simulink model "Model_14Bus_Microgrid_R2018"  (R2018b)
settings: Solver=ode23tb  StartTime=0.0  StopTime=0.35  MaxStep=1e-2  RelTol=1e-3
InitFcn:
  | Set_parameters_R2018
StopFcn:
  | Save_Data;
  | Graphics;
values from neighbouring files (symbols this model uses):
  Clink = Ceq*2    (= 0.217013888889)    [Set_parameters_R2017b.m]    (also in Set_parameters_R2018.m)
  dis1 = 0.15    [Set_parameters_R2017b.m]    (also in Set_parameters_R2018.m)
  dis10 = 6    [Set_parameters_R2017b.m]    (also in Set_parameters_R2018.m)
  dis11 = 3    [Set_parameters_R2017b.m]    (also in Set_parameters_R2018.m)
  dis12 = 6    [Set_parameters_R2017b.m]    (also in Set_parameters_R2018.m)
  dis13 = 3    [Set_parameters_R2017b.m]    (also in Set_parameters_R2018.m)
  dis14 = 2    [Set_parameters_R2017b.m]    (also in Set_parameters_R2018.m)
  dis2 = 0.2    [Set_parameters_R2017b.m]    (also in Set_parameters_R2018.m)
  dis3 = 0.15    [Set_parameters_R2017b.m]    (also in Set_parameters_R2018.m)
  dis4 = 0.4    [Set_parameters_R2017b.m]    (also in Set_parameters_R2018.m)
  dis5 = 0.4    [Set_parameters_R2017b.m]    (also in Set_parameters_R2018.m)
  dis6 = 0.4    [Set_parameters_R2017b.m]    (also in Set_parameters_R2018.m)
  dis7 = 0.1    [Set_parameters_R2017b.m]    (also in Set_parameters_R2018.m)
  dis8 = 2    [Set_parameters_R2017b.m]    (also in Set_parameters_R2018.m)
  dis9 = 6    [Set_parameters_R2017b.m]    (also in Set_parameters_R2018.m)
  Fc = 33 * Fnom    (= 1980)    [Set_parameters_R2017b.m]    (also in Set_parameters_R2018.m)
  Fnom = 60    [Main_DC_MG.m]    (also in Set_parameters_R2017b.m; Set_parameters_R2018.m)
  Increment_MPPT = 0.01    [Set_parameters_R2017b.m]    (also in Set_parameters_R2018.m)
  Ki_Ireg = 20    [Set_parameters_R2017b.m]    (also in Set_parameters_R2018.m)
  Ki_VDCreg = 400    [Set_parameters_R2017b.m]    (also in Set_parameters_R2018.m)
  Kp_Ireg = 0.3    [Set_parameters_R2017b.m]    (also in Set_parameters_R2018.m)
  Kp_VDCreg = 2    [Set_parameters_R2017b.m]    (also in Set_parameters_R2018.m)
  LimitL_Ireg = -1.5    [Set_parameters_R2017b.m]    (also in Set_parameters_R2018.m)
  LimitL_VDCreg = -1.5    [Set_parameters_R2017b.m]    (also in Set_parameters_R2018.m)
  Limits_MPPT = [ 583 357 ]    [Set_parameters_R2017b.m]    (also in Set_parameters_R2018.m)
  LimitU_Ireg = 1.5    [Set_parameters_R2017b.m]    (also in Set_parameters_R2018.m)
  LimitU_VDCreg = 1.5    [Set_parameters_R2017b.m]    (also in Set_parameters_R2018.m)
  P_Load_2 = S_Load_2* PF_Load_2    (= 36000)    [Set_parameters_R2017b.m]    (also in Set_parameters_R2018.m)
  P_Load_3 = S_Load_3* PF_Load_3    (= 25500)    [Set_parameters_R2017b.m]    (also in Set_parameters_R2018.m)
  Pnom = 1e6    (= 1000000)    [Set_parameters_R2017b.m]    (also in Set_parameters_R2018.m)
  Pnom_T1 = 1.5e6    (= 1500000)    [Set_parameters_R2017b.m]    (also in Set_parameters_R2018.m)
  Pnom_T2 = 1.5e6    (= 1500000)    [Set_parameters_R2017b.m]    (also in Set_parameters_R2018.m)
  Pnom_T3 = 4e6    (= 4000000)    [Set_parameters_R2017b.m]    (also in Set_parameters_R2018.m)
  Pnom_xfo = Pnom    (= 1000000)    [Set_parameters_R2017b.m]    (also in Set_parameters_R2018.m)
  Ql_Load_2 = S_Load_2 * sin(acos(PF_Load_2))    [Set_parameters_R2017b.m]    (also in Set_parameters_R2018.m)
  Ql_Load_3 = S_Load_3 * sin(acos(PF_Load_3))    [Set_parameters_R2017b.m]    (also in Set_parameters_R2018.m)
  R_Load_9 = (Vnom_prim * 1.35)^2 / P_Load_9    (= 1084.6153125)    [Set_parameters_R2017b.m]    (also in Set_parameters_R2018.m)
  R_Load_DC = Vnom_DC^2/ P_Load_DC    (= 45)    [Main_DC_MG.m]    (also in Set_parameters_R2017b.m; Set_parameters_R2018.m)
  Rl = 0.394    [Set_parameters_R2017b.m]    (also in Set_parameters_R2018.m)
  Rls = 0.198    [Set_parameters_R2017b.m]    (also in Set_parameters_R2018.m)
  Ts = Ts_Power    (= 5.05050505051e-06)    [Main_DC_MG.m]    (also in Set_parameters_R2017b.m; Set_parameters_R2018.m)
  Ts_Control = 10*Ts_Power    (= 5.05050505051e-05)    [Main_DC_MG.m]    (also in Set_parameters_R2017b.m; Set_parameters_R2018.m)
  Ts_Power = 1/(33*Fnom)/100    (= 5.05050505051e-06)    [Main_DC_MG.m]    (also in Set_parameters_R2017b.m; Set_parameters_R2018.m)
  V1_LL_T3 = 69e3    (= 69000)    [Set_parameters_R2017b.m]    (also in Set_parameters_R2018.m)
  Vf = 0    [Set_parameters_R2017b.m]    (also in Set_parameters_R2018.m)
  Vfd = 0    [Set_parameters_R2017b.m]    (also in Set_parameters_R2018.m)
  Vnom_DC = 300    [Main_DC_MG.m]    (also in Set_parameters_R2017b.m; Set_parameters_R2018.m)
  Vnom_dc = 480    [Set_parameters_R2017b.m]    (also in Set_parameters_R2018.m)
  Vnom_Diesel = 2.4e3    (= 2400)    [Set_parameters_R2017b.m]    (also in Set_parameters_R2018.m)
  Vnom_prim = 13.8e3    (= 13800)    [Set_parameters_R2017b.m]    (also in Set_parameters_R2018.m)
  Vnom_sec = 220    [Set_parameters_R2017b.m]    (also in Set_parameters_R2018.m)
  Vnom_ter_AC_DC = 150    [Set_parameters_R2017b.m]    (also in Set_parameters_R2018.m)
  Xl = 0.1168    [Set_parameters_R2017b.m]    (also in Set_parameters_R2018.m)
  Xls = 0.1089    [Set_parameters_R2017b.m]    (also in Set_parameters_R2018.m)
undefined symbols (not defined in the file or in its folder): D1, Delta, Hydride, Ion, Lithium, max_min, Metal, Nickel, RL, RLff, sigbuilder_block
libraries: powerlib x202, powerlib_meascontrol x152, simulink x14, powerlib_extras x14, electricdrivelib x4, re_lib x2
(part 7 of 10)

== system Model_14Bus_Microgrid_R2018/Load_1/Power Factor Block1 ==
  Vabc : Inport
  Iabc : Inport  Port=2
  Complex to Magnitude-Angle : ComplexToMagnitudeAngle
  Mux : Mux  Inputs=2
  Mux1 : Mux  Inputs=2
  Power : powerlib_meascontrol/Measurements/Power  Freq=Freq  Vinit=Vinit  Iinit=Iinit  Ts=Ts
      settings: SourceProductName=Simscape Electrical
  RMS3 : powerlib_meascontrol/Measurements/RMS  TrueRMS=on  Freq=60  RMSInit=0  Ts=0
      settings: SourceProductName=Simscape Electrical
  RMS4 : powerlib_meascontrol/Measurements/RMS  TrueRMS=on  Freq=60  RMSInit=0  Ts=0
      settings: SourceProductName=Simscape Electrical
  Real-Imag to Complex : RealImagToComplex
  Terminator : Terminator
  compara : Gain  SaturateOnIntegerOverflow=on  OutDataTypeStr=Inherit: Same as input  ParamDataTypeStr=Inherit: Same as input
  cos(theta) : Trigonometry  Operator=cos
  Pabc : Outport
  Qabc : Outport  Port=2
  Vabc y Vabc (rms) : Outport  Port=3
  Iabc y Iabc (rms) : Outport  Port=4
  "PFabc " : Outport  Port=5
  wires:
  Power/1 -> Pabc/1, Real-Imag to Complex/1
  Power/2 -> Qabc/1, Real-Imag to Complex/2
  Complex to Magnitude-Angle/2 -> cos(theta)/1
  Real-Imag to Complex/1 -> Complex to Magnitude-Angle/1
  cos(theta)/1 -> "PFabc "/1
  Complex to Magnitude-Angle/1 -> Terminator/1
  Iabc/1 -> RMS4/1, compara/1, Power/2
  RMS4/1 -> Mux1/2
  Mux1/1 -> Iabc y Iabc (rms)/1
  Mux/1 -> Vabc y Vabc (rms)/1
  Vabc/1 -> Power/1, Mux/2, RMS3/1
  compara/1 -> Mux1/1
  RMS3/1 -> Mux/1

== system Model_14Bus_Microgrid_R2018/Load_2/Power Factor Block1 ==
  Vabc : Inport
  Iabc : Inport  Port=2
  Complex to Magnitude-Angle : ComplexToMagnitudeAngle
  Mux : Mux  Inputs=2
  Mux1 : Mux  Inputs=2
  Power : powerlib_meascontrol/Measurements/Power  Freq=Freq  Vinit=Vinit  Iinit=Iinit  Ts=Ts
      settings: SourceProductName=Simscape Electrical
  RMS3 : powerlib_meascontrol/Measurements/RMS  TrueRMS=on  Freq=60  RMSInit=0  Ts=0
      settings: SourceProductName=Simscape Electrical
  RMS4 : powerlib_meascontrol/Measurements/RMS  TrueRMS=on  Freq=60  RMSInit=0  Ts=0
      settings: SourceProductName=Simscape Electrical
  Real-Imag to Complex : RealImagToComplex
  Terminator : Terminator
  compara : Gain  SaturateOnIntegerOverflow=on  OutDataTypeStr=Inherit: Same as input  ParamDataTypeStr=Inherit: Same as input
  cos(theta) : Trigonometry  Operator=cos
  Pabc : Outport
  Qabc : Outport  Port=2
  Vabc y Vabc (rms) : Outport  Port=3
  Iabc y Iabc (rms) : Outport  Port=4
  "PFabc " : Outport  Port=5
  wires:
  Power/1 -> Pabc/1, Real-Imag to Complex/1
  Power/2 -> Qabc/1, Real-Imag to Complex/2
  Complex to Magnitude-Angle/2 -> cos(theta)/1
  Real-Imag to Complex/1 -> Complex to Magnitude-Angle/1
  cos(theta)/1 -> "PFabc "/1
  Complex to Magnitude-Angle/1 -> Terminator/1
  Iabc/1 -> RMS4/1, compara/1, Power/2
  RMS4/1 -> Mux1/2
  Mux1/1 -> Iabc y Iabc (rms)/1
  Mux/1 -> Vabc y Vabc (rms)/1
  Vabc/1 -> Power/1, Mux/2, RMS3/1
  compara/1 -> Mux1/1
  RMS3/1 -> Mux/1

== system Model_14Bus_Microgrid_R2018/Load_3/Power Factor Block1 ==
  Vabc : Inport
  Iabc : Inport  Port=2
  Complex to Magnitude-Angle : ComplexToMagnitudeAngle
  Mux : Mux  Inputs=2
  Mux1 : Mux  Inputs=2
  Power : powerlib_meascontrol/Measurements/Power  Freq=Freq  Vinit=Vinit  Iinit=Iinit  Ts=Ts
      settings: SourceProductName=Simscape Electrical
  RMS3 : powerlib_meascontrol/Measurements/RMS  TrueRMS=on  Freq=60  RMSInit=0  Ts=0
      settings: SourceProductName=Simscape Electrical
  RMS4 : powerlib_meascontrol/Measurements/RMS  TrueRMS=on  Freq=60  RMSInit=0  Ts=0
      settings: SourceProductName=Simscape Electrical
  Real-Imag to Complex : RealImagToComplex
  Terminator : Terminator
  compara : Gain  SaturateOnIntegerOverflow=on  OutDataTypeStr=Inherit: Same as input  ParamDataTypeStr=Inherit: Same as input
  cos(theta) : Trigonometry  Operator=cos
  Pabc : Outport
  Qabc : Outport  Port=2
  Vabc y Vabc (rms) : Outport  Port=3
  Iabc y Iabc (rms) : Outport  Port=4
  "PFabc " : Outport  Port=5
  wires:
  Power/1 -> Pabc/1, Real-Imag to Complex/1
  Power/2 -> Qabc/1, Real-Imag to Complex/2
  Complex to Magnitude-Angle/2 -> cos(theta)/1
  Real-Imag to Complex/1 -> Complex to Magnitude-Angle/1
  cos(theta)/1 -> "PFabc "/1
  Complex to Magnitude-Angle/1 -> Terminator/1
  Iabc/1 -> RMS4/1, compara/1, Power/2
  RMS4/1 -> Mux1/2
  Mux1/1 -> Iabc y Iabc (rms)/1
  Mux/1 -> Vabc y Vabc (rms)/1
  Vabc/1 -> Power/1, Mux/2, RMS3/1
  compara/1 -> Mux1/1
  RMS3/1 -> Mux/1

== system Model_14Bus_Microgrid_R2018/Load_4/Power Factor Block1 ==
  Vabc : Inport
  Iabc : Inport  Port=2
  Complex to Magnitude-Angle : ComplexToMagnitudeAngle
  Mux : Mux  Inputs=2
  Mux1 : Mux  Inputs=2
  Power : powerlib_meascontrol/Measurements/Power  Freq=Freq  Vinit=Vinit  Iinit=Iinit  Ts=Ts
      settings: SourceProductName=Simscape Electrical
  RMS3 : powerlib_meascontrol/Measurements/RMS  TrueRMS=on  Freq=60  RMSInit=0  Ts=0
      settings: SourceProductName=Simscape Electrical
  RMS4 : powerlib_meascontrol/Measurements/RMS  TrueRMS=on  Freq=60  RMSInit=0  Ts=0
      settings: SourceProductName=Simscape Electrical
  Real-Imag to Complex : RealImagToComplex
  Terminator : Terminator
  compara : Gain  SaturateOnIntegerOverflow=on  OutDataTypeStr=Inherit: Same as input  ParamDataTypeStr=Inherit: Same as input
  cos(theta) : Trigonometry  Operator=cos
  Pabc : Outport
  Qabc : Outport  Port=2
  Vabc y Vabc (rms) : Outport  Port=3
  Iabc y Iabc (rms) : Outport  Port=4
  "PFabc " : Outport  Port=5
  wires:
  Power/1 -> Pabc/1, Real-Imag to Complex/1
  Power/2 -> Qabc/1, Real-Imag to Complex/2
  Complex to Magnitude-Angle/2 -> cos(theta)/1
  Real-Imag to Complex/1 -> Complex to Magnitude-Angle/1
  cos(theta)/1 -> "PFabc "/1
  Complex to Magnitude-Angle/1 -> Terminator/1
  Iabc/1 -> RMS4/1, compara/1, Power/2
  RMS4/1 -> Mux1/2
  Mux1/1 -> Iabc y Iabc (rms)/1
  Mux/1 -> Vabc y Vabc (rms)/1
  Vabc/1 -> Power/1, Mux/2, RMS3/1
  compara/1 -> Mux1/1
  RMS3/1 -> Mux/1

== system Model_14Bus_Microgrid_R2018/Resource1/Irradiance Temp Demand Max ==
  Demux : Demux  Tag=STV Demux  Outputs=2
  FromWs : FromWorkspace  Tag=STV FromWs  VariableName=tuvar  SampleTime=0
      SigBuilderData=|
      | common.afterFinalStr = 'Extrapolate'
      | common.sampleTime = '0'
      | dataSet(1).timeRange = [0 2]
      | dataSet(1).name = 'Constant Irradiance'
      | dataSet(2).timeRange = [0 2]
      | dataSet(2).name = 'Step Irradiance'
      | dataSet(3).timeRange = [0 3]
      | dataSet(3).name = 'Ramp-up/down Irradiance'
      | sbobj.Groups(1).Name = 'Constant Irradiance'
      | sbobj.Groups(1).Signals(1).Name = 'Ir'
      | sbobj.Groups(1).Signals(1).XData = [0 2]
      | sbobj.Groups(1).Signals(1).YData = [1000 1000]
      | sbobj.Groups(1).Signals(2).Name = 'Temp'
      | sbobj.Groups(1).Signals(2).XData = [0 1 1 2]
      | sbobj.Groups(1).Signals(2).YData = [0 0 1 1]
      | sbobj.Groups(1).TimeRange = [0 2]
      | sbobj.Groups(2).Name = 'Step Irradiance'
      | sbobj.Groups(2).Signals(1).Name = 'Ir'
      | sbobj.Groups(2).Signals(1).XData = [0 0.252 0.252 2]
      | sbobj.Groups(2).Signals(1).YData = [600 600 1000 1000]
      | sbobj.Groups(2).Signals(2).Name = 'Temp'
      | sbobj.Groups(2).Signals(2).XData = [0 1 1 2]
      | sbobj.Groups(2).Signals(2).YData = [0 0 1 1]
      | sbobj.Groups(2).TimeRange = [0 2]
      | sbobj.Groups(3).Name = 'Ramp-up/down Irradiance'
      | sbobj.Groups(3).Signals(1).Name = 'Ir'
      | sbobj.Groups(3).Signals(1).XData = [0 0.785 1.7 2.28 3]
      | sbobj.Groups(3).Signals(1).YData = [1000 999.538235294 999 999.446153846 1000]
      | sbobj.Groups(3).Signals(2).Name = 'Temp'
      | sbobj.Groups(3).Signals(2).XData = [0 2 2.1 3]
      | sbobj.Groups(3).Signals(2).YData = [25 25 25 25]
      | sbobj.Groups(3).TimeRange = [0 3]
  Ir : Outport  Tag=STV Outport
  Temp : Outport  Tag=STV Outport  Port=2
  wires:
  Demux/1 -> Ir/1
  FromWs/1 -> Demux/1
  Demux/2 -> Temp/1

== system Model_14Bus_Microgrid_R2018/Resources/Irradiance Temp Demand Max ==
  Demux : Demux  Tag=STV Demux  Outputs=2
  FromWs : FromWorkspace  Tag=STV FromWs  VariableName=tuvar  SampleTime=0
      SigBuilderData=|
      | common.afterFinalStr = 'Extrapolate'
      | common.sampleTime = '0'
      | dataSet(1).timeRange = [0 2]
      | dataSet(1).name = 'Constant Irradiance'
      | dataSet(2).timeRange = [0 2]
      | dataSet(2).name = 'Step Irradiance'
      | dataSet(3).timeRange = [0 3]
      | dataSet(3).name = 'Ramp-up/down Irradiance'
      | sbobj.Groups(1).Name = 'Constant Irradiance'
      | sbobj.Groups(1).Signals(1).Name = 'Ir'
      | sbobj.Groups(1).Signals(1).XData = [0 2]
      | sbobj.Groups(1).Signals(1).YData = [1000 1000]
      | sbobj.Groups(1).Signals(2).Name = 'Temp'
      | sbobj.Groups(1).Signals(2).XData = [0 1 1 2]
      | sbobj.Groups(1).Signals(2).YData = [0 0 1 1]
      | sbobj.Groups(1).TimeRange = [0 2]
      | sbobj.Groups(2).Name = 'Step Irradiance'
      | sbobj.Groups(2).Signals(1).Name = 'Ir'
      | sbobj.Groups(2).Signals(1).XData = [0 0.252 0.252 2]
      | sbobj.Groups(2).Signals(1).YData = [600 600 1000 1000]
      | sbobj.Groups(2).Signals(2).Name = 'Temp'
      | sbobj.Groups(2).Signals(2).XData = [0 1 1 2]
      | sbobj.Groups(2).Signals(2).YData = [0 0 1 1]
      | sbobj.Groups(2).TimeRange = [0 2]
      | sbobj.Groups(3).Name = 'Ramp-up/down Irradiance'
      | sbobj.Groups(3).Signals(1).Name = 'Ir'
      | sbobj.Groups(3).Signals(1).XData = [0 0.785 1.7 2.28 3]
      | sbobj.Groups(3).Signals(1).YData = [1000 999.538235294 999 999.446153846 1000]
      | sbobj.Groups(3).Signals(2).Name = 'Temp'
      | sbobj.Groups(3).Signals(2).XData = [0 2 2.1 3]
      | sbobj.Groups(3).Signals(2).YData = [25 25 25 25]
      | sbobj.Groups(3).TimeRange = [0 3]
  Ir : Outport  Tag=STV Outport
  Temp : Outport  Tag=STV Outport  Port=2
  wires:
  Demux/1 -> Ir/1
  FromWs/1 -> Demux/1
  Demux/2 -> Temp/1

== system Model_14Bus_Microgrid_R2018/Bus_1/PLL/Pll1 ==
  note: error
  note: d'
  note: Fundamental
  note: fase
      | total
  note: fase de la señal
  note: adelanta 90
  note: Este PLL calcula la fase respecto a una onda coseno
  señal : Inport
  w : Inport  Port=2
  Gain : Gain  Gain=-1  SaturateOnIntegerOverflow=on  OutDataTypeStr=Inherit: Same as input  ParamDataTypeStr=Inherit: Same as input
  Integrator : Integrator  InitialCondition=2*pi*60
  Integrator1 : Integrator  InitialCondition=2*pi*60
  Integrator2 : Integrator
  K : Gain  Gain=100  SaturateOnIntegerOverflow=on  OutDataTypeStr=Inherit: Same as input  ParamDataTypeStr=Inherit: Same as input
  Kp : Gain  Gain=10  SaturateOnIntegerOverflow=on  OutDataTypeStr=Inherit: Same as input  ParamDataTypeStr=Inherit: Same as input
  Kp1 : Gain  Gain=10  SaturateOnIntegerOverflow=on  OutDataTypeStr=Inherit: Same as input  ParamDataTypeStr=Inherit: Same as input
  Poduct : Product  SaturateOnIntegerOverflow=on  OutDataTypeStr=Inherit: Same as first input
  Poduct1 : Product  SaturateOnIntegerOverflow=on  OutDataTypeStr=Inherit: Same as first input
  Poduct2 : Product  SaturateOnIntegerOverflow=on  OutDataTypeStr=Inherit: Same as first input
  Sum : Sum  Inputs=|+-  SaturateOnIntegerOverflow=on
  Sum1 : Sum  SaturateOnIntegerOverflow=on
  Sum2 : Sum  Inputs=|-+  SaturateOnIntegerOverflow=on
  Trigonometric Function : Trigonometry
  Trigonometric Function1 : Trigonometry  Operator=cos
  f cos (rad) : Outport
  wires:
  Sum/1 -> Poduct/1, Poduct1/1
  Poduct/1 -> Kp/1
  Kp/1 -> Kp1/1
  Poduct2/1 -> Sum/2
  Trigonometric Function1/1 -> Poduct1/2, Poduct2/1
  Poduct1/1 -> K/1
  K/1 -> Integrator2/1
  Integrator2/1 -> Poduct2/2
  Integrator/1 -> Trigonometric Function/1, Sum2/2, Trigonometric Function1/1
  Integrator1/1 -> Sum2/1
  Sum2/1 -> f cos (rad)/1
  w/1 -> Sum1/1, Integrator1/1
  Kp1/1 -> Sum1/2
  Sum1/1 -> Integrator/1
  Trigonometric Function/1 -> Gain/1
  Gain/1 -> Poduct/2
  señal/1 -> Sum/1

== system Model_14Bus_Microgrid_R2018/Bus_1/PLL/Pll2 ==
  note: error
  note: d'
  note: Fundamental
  note: fase
      | total
  note: fase de la señal
  note: adelanta 90
  note: Este PLL calcula la fase respecto a una onda coseno
  señal : Inport
  w : Inport  Port=2
  Gain : Gain  Gain=-1  SaturateOnIntegerOverflow=on  OutDataTypeStr=Inherit: Same as input  ParamDataTypeStr=Inherit: Same as input
  Integrator : Integrator  InitialCondition=2*pi*60
  Integrator1 : Integrator  InitialCondition=2*pi*60
  Integrator2 : Integrator
  K : Gain  Gain=100  SaturateOnIntegerOverflow=on  OutDataTypeStr=Inherit: Same as input  ParamDataTypeStr=Inherit: Same as input
  Kp : Gain  Gain=10  SaturateOnIntegerOverflow=on  OutDataTypeStr=Inherit: Same as input  ParamDataTypeStr=Inherit: Same as input
  Kp1 : Gain  Gain=10  SaturateOnIntegerOverflow=on  OutDataTypeStr=Inherit: Same as input  ParamDataTypeStr=Inherit: Same as input
  Poduct : Product  SaturateOnIntegerOverflow=on  OutDataTypeStr=Inherit: Same as first input
  Poduct1 : Product  SaturateOnIntegerOverflow=on  OutDataTypeStr=Inherit: Same as first input
  Poduct2 : Product  SaturateOnIntegerOverflow=on  OutDataTypeStr=Inherit: Same as first input
  Sum : Sum  Inputs=|+-  SaturateOnIntegerOverflow=on
  Sum1 : Sum  SaturateOnIntegerOverflow=on
  Sum2 : Sum  Inputs=|-+  SaturateOnIntegerOverflow=on
  Trigonometric Function : Trigonometry
  Trigonometric Function1 : Trigonometry  Operator=cos
  f cos (rad) : Outport
  wires:
  Sum/1 -> Poduct/1, Poduct1/1
  Poduct/1 -> Kp/1
  Kp/1 -> Kp1/1
  Poduct2/1 -> Sum/2
  Trigonometric Function1/1 -> Poduct1/2, Poduct2/1
  Poduct1/1 -> K/1
  K/1 -> Integrator2/1
  Integrator2/1 -> Poduct2/2
  Integrator/1 -> Trigonometric Function/1, Sum2/2, Trigonometric Function1/1
  Integrator1/1 -> Sum2/1
  Sum2/1 -> f cos (rad)/1
  w/1 -> Sum1/1, Integrator1/1
  Kp1/1 -> Sum1/2
  Sum1/1 -> Integrator/1
  Trigonometric Function/1 -> Gain/1
  Gain/1 -> Poduct/2
  señal/1 -> Sum/1

== system Model_14Bus_Microgrid_R2018/Bus_1/PLL/Pll3 ==
  note: error
  note: d'
  note: Fundamental
  note: fase
      | total
  note: fase de la señal
  note: adelanta 90
  note: Este PLL calcula la fase respecto a una onda coseno
  señal : Inport
  w : Inport  Port=2
  Gain : Gain  Gain=-1  SaturateOnIntegerOverflow=on  OutDataTypeStr=Inherit: Same as input  ParamDataTypeStr=Inherit: Same as input
  Integrator : Integrator  InitialCondition=2*pi*60
  Integrator1 : Integrator  InitialCondition=2*pi*60
  Integrator2 : Integrator
  K : Gain  Gain=100  SaturateOnIntegerOverflow=on  OutDataTypeStr=Inherit: Same as input  ParamDataTypeStr=Inherit: Same as input
  Kp : Gain  Gain=10  SaturateOnIntegerOverflow=on  OutDataTypeStr=Inherit: Same as input  ParamDataTypeStr=Inherit: Same as input
  Kp1 : Gain  Gain=10  SaturateOnIntegerOverflow=on  OutDataTypeStr=Inherit: Same as input  ParamDataTypeStr=Inherit: Same as input
  Poduct : Product  SaturateOnIntegerOverflow=on  OutDataTypeStr=Inherit: Same as first input
  Poduct1 : Product  SaturateOnIntegerOverflow=on  OutDataTypeStr=Inherit: Same as first input
  Poduct2 : Product  SaturateOnIntegerOverflow=on  OutDataTypeStr=Inherit: Same as first input
  Sum : Sum  Inputs=|+-  SaturateOnIntegerOverflow=on
  Sum1 : Sum  SaturateOnIntegerOverflow=on
  Sum2 : Sum  Inputs=|-+  SaturateOnIntegerOverflow=on
  Trigonometric Function : Trigonometry
  Trigonometric Function1 : Trigonometry  Operator=cos
  f cos (rad) : Outport
  wires:
  Sum/1 -> Poduct/1, Poduct1/1
  Poduct/1 -> Kp/1
  Kp/1 -> Kp1/1
  Poduct2/1 -> Sum/2
  Trigonometric Function1/1 -> Poduct1/2, Poduct2/1
  Poduct1/1 -> K/1
  K/1 -> Integrator2/1
  Integrator2/1 -> Poduct2/2
  Integrator/1 -> Trigonometric Function/1, Sum2/2, Trigonometric Function1/1
  Integrator1/1 -> Sum2/1
  Sum2/1 -> f cos (rad)/1
  w/1 -> Sum1/1, Integrator1/1
  Kp1/1 -> Sum1/2
  Sum1/1 -> Integrator/1
  Trigonometric Function/1 -> Gain/1
  Gain/1 -> Poduct/2
  señal/1 -> Sum/1

== system Model_14Bus_Microgrid_R2018/Bus_10/PLL/Pll1 ==
  note: error
  note: d'
  note: Fundamental
  note: fase
      | total
  note: fase de la señal
  note: adelanta 90
  note: Este PLL calcula la fase respecto a una onda coseno
  señal : Inport
  w : Inport  Port=2
  Gain : Gain  Gain=-1  SaturateOnIntegerOverflow=on  OutDataTypeStr=Inherit: Same as input  ParamDataTypeStr=Inherit: Same as input
  Integrator : Integrator  InitialCondition=2*pi*60
  Integrator1 : Integrator  InitialCondition=2*pi*60
  Integrator2 : Integrator
  K : Gain  Gain=100  SaturateOnIntegerOverflow=on  OutDataTypeStr=Inherit: Same as input  ParamDataTypeStr=Inherit: Same as input
  Kp : Gain  Gain=10  SaturateOnIntegerOverflow=on  OutDataTypeStr=Inherit: Same as input  ParamDataTypeStr=Inherit: Same as input
  Kp1 : Gain  Gain=10  SaturateOnIntegerOverflow=on  OutDataTypeStr=Inherit: Same as input  ParamDataTypeStr=Inherit: Same as input
  Poduct : Product  SaturateOnIntegerOverflow=on  OutDataTypeStr=Inherit: Same as first input
  Poduct1 : Product  SaturateOnIntegerOverflow=on  OutDataTypeStr=Inherit: Same as first input
  Poduct2 : Product  SaturateOnIntegerOverflow=on  OutDataTypeStr=Inherit: Same as first input
  Sum : Sum  Inputs=|+-  SaturateOnIntegerOverflow=on
  Sum1 : Sum  SaturateOnIntegerOverflow=on
  Sum2 : Sum  Inputs=|-+  SaturateOnIntegerOverflow=on
  Trigonometric Function : Trigonometry
  Trigonometric Function1 : Trigonometry  Operator=cos
  f cos (rad) : Outport
  wires:
  Sum/1 -> Poduct/1, Poduct1/1
  Poduct/1 -> Kp/1
  Kp/1 -> Kp1/1
  Poduct2/1 -> Sum/2
  Trigonometric Function1/1 -> Poduct1/2, Poduct2/1
  Poduct1/1 -> K/1
  K/1 -> Integrator2/1
  Integrator2/1 -> Poduct2/2
  Integrator/1 -> Trigonometric Function/1, Sum2/2, Trigonometric Function1/1
  Integrator1/1 -> Sum2/1
  Sum2/1 -> f cos (rad)/1
  w/1 -> Sum1/1, Integrator1/1
  Kp1/1 -> Sum1/2
  Sum1/1 -> Integrator/1
  Trigonometric Function/1 -> Gain/1
  Gain/1 -> Poduct/2
  señal/1 -> Sum/1

== system Model_14Bus_Microgrid_R2018/Bus_10/PLL/Pll2 ==
  note: error
  note: d'
  note: Fundamental
  note: fase
      | total
  note: fase de la señal
  note: adelanta 90
  note: Este PLL calcula la fase respecto a una onda coseno
  señal : Inport
  w : Inport  Port=2
  Gain : Gain  Gain=-1  SaturateOnIntegerOverflow=on  OutDataTypeStr=Inherit: Same as input  ParamDataTypeStr=Inherit: Same as input
  Integrator : Integrator  InitialCondition=2*pi*60
  Integrator1 : Integrator  InitialCondition=2*pi*60
  Integrator2 : Integrator
  K : Gain  Gain=100  SaturateOnIntegerOverflow=on  OutDataTypeStr=Inherit: Same as input  ParamDataTypeStr=Inherit: Same as input
  Kp : Gain  Gain=10  SaturateOnIntegerOverflow=on  OutDataTypeStr=Inherit: Same as input  ParamDataTypeStr=Inherit: Same as input
  Kp1 : Gain  Gain=10  SaturateOnIntegerOverflow=on  OutDataTypeStr=Inherit: Same as input  ParamDataTypeStr=Inherit: Same as input
  Poduct : Product  SaturateOnIntegerOverflow=on  OutDataTypeStr=Inherit: Same as first input
  Poduct1 : Product  SaturateOnIntegerOverflow=on  OutDataTypeStr=Inherit: Same as first input
  Poduct2 : Product  SaturateOnIntegerOverflow=on  OutDataTypeStr=Inherit: Same as first input
  Sum : Sum  Inputs=|+-  SaturateOnIntegerOverflow=on
  Sum1 : Sum  SaturateOnIntegerOverflow=on
  Sum2 : Sum  Inputs=|-+  SaturateOnIntegerOverflow=on
  Trigonometric Function : Trigonometry
  Trigonometric Function1 : Trigonometry  Operator=cos
  f cos (rad) : Outport
  wires:
  Sum/1 -> Poduct/1, Poduct1/1
  Poduct/1 -> Kp/1
  Kp/1 -> Kp1/1
  Poduct2/1 -> Sum/2
  Trigonometric Function1/1 -> Poduct1/2, Poduct2/1
  Poduct1/1 -> K/1
  K/1 -> Integrator2/1
  Integrator2/1 -> Poduct2/2
  Integrator/1 -> Trigonometric Function/1, Sum2/2, Trigonometric Function1/1
  Integrator1/1 -> Sum2/1
  Sum2/1 -> f cos (rad)/1
  w/1 -> Sum1/1, Integrator1/1
  Kp1/1 -> Sum1/2
  Sum1/1 -> Integrator/1
  Trigonometric Function/1 -> Gain/1
  Gain/1 -> Poduct/2
  señal/1 -> Sum/1

== system Model_14Bus_Microgrid_R2018/Bus_10/PLL/Pll3 ==
  note: error
  note: d'
  note: Fundamental
  note: fase
      | total
  note: fase de la señal
  note: adelanta 90
  note: Este PLL calcula la fase respecto a una onda coseno
  señal : Inport
  w : Inport  Port=2
  Gain : Gain  Gain=-1  SaturateOnIntegerOverflow=on  OutDataTypeStr=Inherit: Same as input  ParamDataTypeStr=Inherit: Same as input
  Integrator : Integrator  InitialCondition=2*pi*60
  Integrator1 : Integrator  InitialCondition=2*pi*60
  Integrator2 : Integrator
  K : Gain  Gain=100  SaturateOnIntegerOverflow=on  OutDataTypeStr=Inherit: Same as input  ParamDataTypeStr=Inherit: Same as input
  Kp : Gain  Gain=10  SaturateOnIntegerOverflow=on  OutDataTypeStr=Inherit: Same as input  ParamDataTypeStr=Inherit: Same as input
  Kp1 : Gain  Gain=10  SaturateOnIntegerOverflow=on  OutDataTypeStr=Inherit: Same as input  ParamDataTypeStr=Inherit: Same as input
  Poduct : Product  SaturateOnIntegerOverflow=on  OutDataTypeStr=Inherit: Same as first input
  Poduct1 : Product  SaturateOnIntegerOverflow=on  OutDataTypeStr=Inherit: Same as first input
  Poduct2 : Product  SaturateOnIntegerOverflow=on  OutDataTypeStr=Inherit: Same as first input
  Sum : Sum  Inputs=|+-  SaturateOnIntegerOverflow=on
  Sum1 : Sum  SaturateOnIntegerOverflow=on
  Sum2 : Sum  Inputs=|-+  SaturateOnIntegerOverflow=on
  Trigonometric Function : Trigonometry
  Trigonometric Function1 : Trigonometry  Operator=cos
  f cos (rad) : Outport
  wires:
  Sum/1 -> Poduct/1, Poduct1/1
  Poduct/1 -> Kp/1
  Kp/1 -> Kp1/1
  Poduct2/1 -> Sum/2
  Trigonometric Function1/1 -> Poduct1/2, Poduct2/1
  Poduct1/1 -> K/1
  K/1 -> Integrator2/1
  Integrator2/1 -> Poduct2/2
  Integrator/1 -> Trigonometric Function/1, Sum2/2, Trigonometric Function1/1
  Integrator1/1 -> Sum2/1
  Sum2/1 -> f cos (rad)/1
  w/1 -> Sum1/1, Integrator1/1
  Kp1/1 -> Sum1/2
  Sum1/1 -> Integrator/1
  Trigonometric Function/1 -> Gain/1
  Gain/1 -> Poduct/2
  señal/1 -> Sum/1

== system Model_14Bus_Microgrid_R2018/Bus_11/PLL/Pll1 ==
  note: error
  note: d'
  note: Fundamental
  note: fase
      | total
  note: fase de la señal
  note: adelanta 90
  note: Este PLL calcula la fase respecto a una onda coseno
  señal : Inport
  w : Inport  Port=2
  Gain : Gain  Gain=-1  SaturateOnIntegerOverflow=on  OutDataTypeStr=Inherit: Same as input  ParamDataTypeStr=Inherit: Same as input
  Integrator : Integrator  InitialCondition=2*pi*60
  Integrator1 : Integrator  InitialCondition=2*pi*60
  Integrator2 : Integrator
  K : Gain  Gain=100  SaturateOnIntegerOverflow=on  OutDataTypeStr=Inherit: Same as input  ParamDataTypeStr=Inherit: Same as input
  Kp : Gain  Gain=10  SaturateOnIntegerOverflow=on  OutDataTypeStr=Inherit: Same as input  ParamDataTypeStr=Inherit: Same as input
  Kp1 : Gain  Gain=10  SaturateOnIntegerOverflow=on  OutDataTypeStr=Inherit: Same as input  ParamDataTypeStr=Inherit: Same as input
  Poduct : Product  SaturateOnIntegerOverflow=on  OutDataTypeStr=Inherit: Same as first input
  Poduct1 : Product  SaturateOnIntegerOverflow=on  OutDataTypeStr=Inherit: Same as first input
  Poduct2 : Product  SaturateOnIntegerOverflow=on  OutDataTypeStr=Inherit: Same as first input
  Sum : Sum  Inputs=|+-  SaturateOnIntegerOverflow=on
  Sum1 : Sum  SaturateOnIntegerOverflow=on
  Sum2 : Sum  Inputs=|-+  SaturateOnIntegerOverflow=on
  Trigonometric Function : Trigonometry
  Trigonometric Function1 : Trigonometry  Operator=cos
  f cos (rad) : Outport
  wires:
  Sum/1 -> Poduct/1, Poduct1/1
  Poduct/1 -> Kp/1
  Kp/1 -> Kp1/1
  Poduct2/1 -> Sum/2
  Trigonometric Function1/1 -> Poduct1/2, Poduct2/1
  Poduct1/1 -> K/1
  K/1 -> Integrator2/1
  Integrator2/1 -> Poduct2/2
  Integrator/1 -> Trigonometric Function/1, Sum2/2, Trigonometric Function1/1
  Integrator1/1 -> Sum2/1
  Sum2/1 -> f cos (rad)/1
  w/1 -> Sum1/1, Integrator1/1
  Kp1/1 -> Sum1/2
  Sum1/1 -> Integrator/1
  Trigonometric Function/1 -> Gain/1
  Gain/1 -> Poduct/2
  señal/1 -> Sum/1

== system Model_14Bus_Microgrid_R2018/Bus_11/PLL/Pll2 ==
  note: error
  note: d'
  note: Fundamental
  note: fase
      | total
  note: fase de la señal
  note: adelanta 90
  note: Este PLL calcula la fase respecto a una onda coseno
  señal : Inport
  w : Inport  Port=2
  Gain : Gain  Gain=-1  SaturateOnIntegerOverflow=on  OutDataTypeStr=Inherit: Same as input  ParamDataTypeStr=Inherit: Same as input
  Integrator : Integrator  InitialCondition=2*pi*60
  Integrator1 : Integrator  InitialCondition=2*pi*60
  Integrator2 : Integrator
  K : Gain  Gain=100  SaturateOnIntegerOverflow=on  OutDataTypeStr=Inherit: Same as input  ParamDataTypeStr=Inherit: Same as input
  Kp : Gain  Gain=10  SaturateOnIntegerOverflow=on  OutDataTypeStr=Inherit: Same as input  ParamDataTypeStr=Inherit: Same as input
  Kp1 : Gain  Gain=10  SaturateOnIntegerOverflow=on  OutDataTypeStr=Inherit: Same as input  ParamDataTypeStr=Inherit: Same as input
  Poduct : Product  SaturateOnIntegerOverflow=on  OutDataTypeStr=Inherit: Same as first input
  Poduct1 : Product  SaturateOnIntegerOverflow=on  OutDataTypeStr=Inherit: Same as first input
  Poduct2 : Product  SaturateOnIntegerOverflow=on  OutDataTypeStr=Inherit: Same as first input
  Sum : Sum  Inputs=|+-  SaturateOnIntegerOverflow=on
  Sum1 : Sum  SaturateOnIntegerOverflow=on
  Sum2 : Sum  Inputs=|-+  SaturateOnIntegerOverflow=on
  Trigonometric Function : Trigonometry
  Trigonometric Function1 : Trigonometry  Operator=cos
  f cos (rad) : Outport
  wires:
  Sum/1 -> Poduct/1, Poduct1/1
  Poduct/1 -> Kp/1
  Kp/1 -> Kp1/1
  Poduct2/1 -> Sum/2
  Trigonometric Function1/1 -> Poduct1/2, Poduct2/1
  Poduct1/1 -> K/1
  K/1 -> Integrator2/1
  Integrator2/1 -> Poduct2/2
  Integrator/1 -> Trigonometric Function/1, Sum2/2, Trigonometric Function1/1
  Integrator1/1 -> Sum2/1
  Sum2/1 -> f cos (rad)/1
  w/1 -> Sum1/1, Integrator1/1
  Kp1/1 -> Sum1/2
  Sum1/1 -> Integrator/1
  Trigonometric Function/1 -> Gain/1
  Gain/1 -> Poduct/2
  señal/1 -> Sum/1

== system Model_14Bus_Microgrid_R2018/Bus_11/PLL/Pll3 ==
  note: error
  note: d'
  note: Fundamental
  note: fase
      | total
  note: fase de la señal
  note: adelanta 90
  note: Este PLL calcula la fase respecto a una onda coseno
  señal : Inport
  w : Inport  Port=2
  Gain : Gain  Gain=-1  SaturateOnIntegerOverflow=on  OutDataTypeStr=Inherit: Same as input  ParamDataTypeStr=Inherit: Same as input
  Integrator : Integrator  InitialCondition=2*pi*60
  Integrator1 : Integrator  InitialCondition=2*pi*60
  Integrator2 : Integrator
  K : Gain  Gain=100  SaturateOnIntegerOverflow=on  OutDataTypeStr=Inherit: Same as input  ParamDataTypeStr=Inherit: Same as input
  Kp : Gain  Gain=10  SaturateOnIntegerOverflow=on  OutDataTypeStr=Inherit: Same as input  ParamDataTypeStr=Inherit: Same as input
  Kp1 : Gain  Gain=10  SaturateOnIntegerOverflow=on  OutDataTypeStr=Inherit: Same as input  ParamDataTypeStr=Inherit: Same as input
  Poduct : Product  SaturateOnIntegerOverflow=on  OutDataTypeStr=Inherit: Same as first input
  Poduct1 : Product  SaturateOnIntegerOverflow=on  OutDataTypeStr=Inherit: Same as first input
  Poduct2 : Product  SaturateOnIntegerOverflow=on  OutDataTypeStr=Inherit: Same as first input
  Sum : Sum  Inputs=|+-  SaturateOnIntegerOverflow=on
  Sum1 : Sum  SaturateOnIntegerOverflow=on
  Sum2 : Sum  Inputs=|-+  SaturateOnIntegerOverflow=on
  Trigonometric Function : Trigonometry
  Trigonometric Function1 : Trigonometry  Operator=cos
  f cos (rad) : Outport
  wires:
  Sum/1 -> Poduct/1, Poduct1/1
  Poduct/1 -> Kp/1
  Kp/1 -> Kp1/1
  Poduct2/1 -> Sum/2
  Trigonometric Function1/1 -> Poduct1/2, Poduct2/1
  Poduct1/1 -> K/1
  K/1 -> Integrator2/1
  Integrator2/1 -> Poduct2/2
  Integrator/1 -> Trigonometric Function/1, Sum2/2, Trigonometric Function1/1
  Integrator1/1 -> Sum2/1
  Sum2/1 -> f cos (rad)/1
  w/1 -> Sum1/1, Integrator1/1
  Kp1/1 -> Sum1/2
  Sum1/1 -> Integrator/1
  Trigonometric Function/1 -> Gain/1
  Gain/1 -> Poduct/2
  señal/1 -> Sum/1

== system Model_14Bus_Microgrid_R2018/Bus_12/PLL/Pll1 ==
  note: error
  note: d'
  note: Fundamental
  note: fase
      | total
  note: fase de la señal
  note: adelanta 90
  note: Este PLL calcula la fase respecto a una onda coseno
  señal : Inport
  w : Inport  Port=2
  Gain : Gain  Gain=-1  SaturateOnIntegerOverflow=on  OutDataTypeStr=Inherit: Same as input  ParamDataTypeStr=Inherit: Same as input
  Integrator : Integrator  InitialCondition=2*pi*60
  Integrator1 : Integrator  InitialCondition=2*pi*60
  Integrator2 : Integrator
  K : Gain  Gain=100  SaturateOnIntegerOverflow=on  OutDataTypeStr=Inherit: Same as input  ParamDataTypeStr=Inherit: Same as input
  Kp : Gain  Gain=10  SaturateOnIntegerOverflow=on  OutDataTypeStr=Inherit: Same as input  ParamDataTypeStr=Inherit: Same as input
  Kp1 : Gain  Gain=10  SaturateOnIntegerOverflow=on  OutDataTypeStr=Inherit: Same as input  ParamDataTypeStr=Inherit: Same as input
  Poduct : Product  SaturateOnIntegerOverflow=on  OutDataTypeStr=Inherit: Same as first input
  Poduct1 : Product  SaturateOnIntegerOverflow=on  OutDataTypeStr=Inherit: Same as first input
  Poduct2 : Product  SaturateOnIntegerOverflow=on  OutDataTypeStr=Inherit: Same as first input
  Sum : Sum  Inputs=|+-  SaturateOnIntegerOverflow=on
  Sum1 : Sum  SaturateOnIntegerOverflow=on
  Sum2 : Sum  Inputs=|-+  SaturateOnIntegerOverflow=on
  Trigonometric Function : Trigonometry
  Trigonometric Function1 : Trigonometry  Operator=cos
  f cos (rad) : Outport
  wires:
  Sum/1 -> Poduct/1, Poduct1/1
  Poduct/1 -> Kp/1
  Kp/1 -> Kp1/1
  Poduct2/1 -> Sum/2
  Trigonometric Function1/1 -> Poduct1/2, Poduct2/1
  Poduct1/1 -> K/1
  K/1 -> Integrator2/1
  Integrator2/1 -> Poduct2/2
  Integrator/1 -> Trigonometric Function/1, Sum2/2, Trigonometric Function1/1
  Integrator1/1 -> Sum2/1
  Sum2/1 -> f cos (rad)/1
  w/1 -> Sum1/1, Integrator1/1
  Kp1/1 -> Sum1/2
  Sum1/1 -> Integrator/1
  Trigonometric Function/1 -> Gain/1
  Gain/1 -> Poduct/2
  señal/1 -> Sum/1

== system Model_14Bus_Microgrid_R2018/Bus_12/PLL/Pll2 ==
  note: error
  note: d'
  note: Fundamental
  note: fase
      | total
  note: fase de la señal
  note: adelanta 90
  note: Este PLL calcula la fase respecto a una onda coseno
  señal : Inport
  w : Inport  Port=2
  Gain : Gain  Gain=-1  SaturateOnIntegerOverflow=on  OutDataTypeStr=Inherit: Same as input  ParamDataTypeStr=Inherit: Same as input
  Integrator : Integrator  InitialCondition=2*pi*60
  Integrator1 : Integrator  InitialCondition=2*pi*60
  Integrator2 : Integrator
  K : Gain  Gain=100  SaturateOnIntegerOverflow=on  OutDataTypeStr=Inherit: Same as input  ParamDataTypeStr=Inherit: Same as input
  Kp : Gain  Gain=10  SaturateOnIntegerOverflow=on  OutDataTypeStr=Inherit: Same as input  ParamDataTypeStr=Inherit: Same as input
  Kp1 : Gain  Gain=10  SaturateOnIntegerOverflow=on  OutDataTypeStr=Inherit: Same as input  ParamDataTypeStr=Inherit: Same as input
  Poduct : Product  SaturateOnIntegerOverflow=on  OutDataTypeStr=Inherit: Same as first input
  Poduct1 : Product  SaturateOnIntegerOverflow=on  OutDataTypeStr=Inherit: Same as first input
  Poduct2 : Product  SaturateOnIntegerOverflow=on  OutDataTypeStr=Inherit: Same as first input
  Sum : Sum  Inputs=|+-  SaturateOnIntegerOverflow=on
  Sum1 : Sum  SaturateOnIntegerOverflow=on
  Sum2 : Sum  Inputs=|-+  SaturateOnIntegerOverflow=on
  Trigonometric Function : Trigonometry
  Trigonometric Function1 : Trigonometry  Operator=cos
  f cos (rad) : Outport
  wires:
  Sum/1 -> Poduct/1, Poduct1/1
  Poduct/1 -> Kp/1
  Kp/1 -> Kp1/1
  Poduct2/1 -> Sum/2
  Trigonometric Function1/1 -> Poduct1/2, Poduct2/1
  Poduct1/1 -> K/1
  K/1 -> Integrator2/1
  Integrator2/1 -> Poduct2/2
  Integrator/1 -> Trigonometric Function/1, Sum2/2, Trigonometric Function1/1
  Integrator1/1 -> Sum2/1
  Sum2/1 -> f cos (rad)/1
  w/1 -> Sum1/1, Integrator1/1
  Kp1/1 -> Sum1/2
  Sum1/1 -> Integrator/1
  Trigonometric Function/1 -> Gain/1
  Gain/1 -> Poduct/2
  señal/1 -> Sum/1

== system Model_14Bus_Microgrid_R2018/Bus_12/PLL/Pll3 ==
  note: error
  note: d'
  note: Fundamental
  note: fase
      | total
  note: fase de la señal
  note: adelanta 90
  note: Este PLL calcula la fase respecto a una onda coseno
  señal : Inport
  w : Inport  Port=2
  Gain : Gain  Gain=-1  SaturateOnIntegerOverflow=on  OutDataTypeStr=Inherit: Same as input  ParamDataTypeStr=Inherit: Same as input
  Integrator : Integrator  InitialCondition=2*pi*60
  Integrator1 : Integrator  InitialCondition=2*pi*60
  Integrator2 : Integrator
  K : Gain  Gain=100  SaturateOnIntegerOverflow=on  OutDataTypeStr=Inherit: Same as input  ParamDataTypeStr=Inherit: Same as input
  Kp : Gain  Gain=10  SaturateOnIntegerOverflow=on  OutDataTypeStr=Inherit: Same as input  ParamDataTypeStr=Inherit: Same as input
  Kp1 : Gain  Gain=10  SaturateOnIntegerOverflow=on  OutDataTypeStr=Inherit: Same as input  ParamDataTypeStr=Inherit: Same as input
  Poduct : Product  SaturateOnIntegerOverflow=on  OutDataTypeStr=Inherit: Same as first input
  Poduct1 : Product  SaturateOnIntegerOverflow=on  OutDataTypeStr=Inherit: Same as first input
  Poduct2 : Product  SaturateOnIntegerOverflow=on  OutDataTypeStr=Inherit: Same as first input
  Sum : Sum  Inputs=|+-  SaturateOnIntegerOverflow=on
  Sum1 : Sum  SaturateOnIntegerOverflow=on
  Sum2 : Sum  Inputs=|-+  SaturateOnIntegerOverflow=on
  Trigonometric Function : Trigonometry
  Trigonometric Function1 : Trigonometry  Operator=cos
  f cos (rad) : Outport
  wires:
  Sum/1 -> Poduct/1, Poduct1/1
  Poduct/1 -> Kp/1
  Kp/1 -> Kp1/1
  Poduct2/1 -> Sum/2
  Trigonometric Function1/1 -> Poduct1/2, Poduct2/1
  Poduct1/1 -> K/1
  K/1 -> Integrator2/1
  Integrator2/1 -> Poduct2/2
  Integrator/1 -> Trigonometric Function/1, Sum2/2, Trigonometric Function1/1
  Integrator1/1 -> Sum2/1
  Sum2/1 -> f cos (rad)/1
  w/1 -> Sum1/1, Integrator1/1
  Kp1/1 -> Sum1/2
  Sum1/1 -> Integrator/1
  Trigonometric Function/1 -> Gain/1
  Gain/1 -> Poduct/2
  señal/1 -> Sum/1

== system Model_14Bus_Microgrid_R2018/Bus_14 /PLL/Pll1 ==
  note: error
  note: d'
  note: Fundamental
  note: fase
      | total
  note: fase de la señal
  note: adelanta 90
  note: Este PLL calcula la fase respecto a una onda coseno
  señal : Inport
  w : Inport  Port=2
  Gain : Gain  Gain=-1  SaturateOnIntegerOverflow=on  OutDataTypeStr=Inherit: Same as input  ParamDataTypeStr=Inherit: Same as input
  Integrator : Integrator  InitialCondition=2*pi*60
  Integrator1 : Integrator  InitialCondition=2*pi*60
  Integrator2 : Integrator
  K : Gain  Gain=100  SaturateOnIntegerOverflow=on  OutDataTypeStr=Inherit: Same as input  ParamDataTypeStr=Inherit: Same as input
  Kp : Gain  Gain=10  SaturateOnIntegerOverflow=on  OutDataTypeStr=Inherit: Same as input  ParamDataTypeStr=Inherit: Same as input
  Kp1 : Gain  Gain=10  SaturateOnIntegerOverflow=on  OutDataTypeStr=Inherit: Same as input  ParamDataTypeStr=Inherit: Same as input
  Poduct : Product  SaturateOnIntegerOverflow=on  OutDataTypeStr=Inherit: Same as first input
  Poduct1 : Product  SaturateOnIntegerOverflow=on  OutDataTypeStr=Inherit: Same as first input
  Poduct2 : Product  SaturateOnIntegerOverflow=on  OutDataTypeStr=Inherit: Same as first input
  Sum : Sum  Inputs=|+-  SaturateOnIntegerOverflow=on
  Sum1 : Sum  SaturateOnIntegerOverflow=on
  Sum2 : Sum  Inputs=|-+  SaturateOnIntegerOverflow=on
  Trigonometric Function : Trigonometry
  Trigonometric Function1 : Trigonometry  Operator=cos
  f cos (rad) : Outport
  wires:
  Sum/1 -> Poduct/1, Poduct1/1
  Poduct/1 -> Kp/1
  Kp/1 -> Kp1/1
  Poduct2/1 -> Sum/2
  Trigonometric Function1/1 -> Poduct1/2, Poduct2/1
  Poduct1/1 -> K/1
  K/1 -> Integrator2/1
  Integrator2/1 -> Poduct2/2
  Integrator/1 -> Trigonometric Function/1, Sum2/2, Trigonometric Function1/1
  Integrator1/1 -> Sum2/1
  Sum2/1 -> f cos (rad)/1
  w/1 -> Sum1/1, Integrator1/1
  Kp1/1 -> Sum1/2
  Sum1/1 -> Integrator/1
  Trigonometric Function/1 -> Gain/1
  Gain/1 -> Poduct/2
  señal/1 -> Sum/1

== system Model_14Bus_Microgrid_R2018/Bus_14 /PLL/Pll2 ==
  note: error
  note: d'
  note: Fundamental
  note: fase
      | total
  note: fase de la señal
  note: adelanta 90
  note: Este PLL calcula la fase respecto a una onda coseno
  señal : Inport
  w : Inport  Port=2
  Gain : Gain  Gain=-1  SaturateOnIntegerOverflow=on  OutDataTypeStr=Inherit: Same as input  ParamDataTypeStr=Inherit: Same as input
  Integrator : Integrator  InitialCondition=2*pi*60
  Integrator1 : Integrator  InitialCondition=2*pi*60
  Integrator2 : Integrator
  K : Gain  Gain=100  SaturateOnIntegerOverflow=on  OutDataTypeStr=Inherit: Same as input  ParamDataTypeStr=Inherit: Same as input
  Kp : Gain  Gain=10  SaturateOnIntegerOverflow=on  OutDataTypeStr=Inherit: Same as input  ParamDataTypeStr=Inherit: Same as input
  Kp1 : Gain  Gain=10  SaturateOnIntegerOverflow=on  OutDataTypeStr=Inherit: Same as input  ParamDataTypeStr=Inherit: Same as input
  Poduct : Product  SaturateOnIntegerOverflow=on  OutDataTypeStr=Inherit: Same as first input
  Poduct1 : Product  SaturateOnIntegerOverflow=on  OutDataTypeStr=Inherit: Same as first input
  Poduct2 : Product  SaturateOnIntegerOverflow=on  OutDataTypeStr=Inherit: Same as first input
  Sum : Sum  Inputs=|+-  SaturateOnIntegerOverflow=on
  Sum1 : Sum  SaturateOnIntegerOverflow=on
  Sum2 : Sum  Inputs=|-+  SaturateOnIntegerOverflow=on
  Trigonometric Function : Trigonometry
  Trigonometric Function1 : Trigonometry  Operator=cos
  f cos (rad) : Outport
  wires:
  Sum/1 -> Poduct/1, Poduct1/1
  Poduct/1 -> Kp/1
  Kp/1 -> Kp1/1
  Poduct2/1 -> Sum/2
  Trigonometric Function1/1 -> Poduct1/2, Poduct2/1
  Poduct1/1 -> K/1
  K/1 -> Integrator2/1
  Integrator2/1 -> Poduct2/2
  Integrator/1 -> Trigonometric Function/1, Sum2/2, Trigonometric Function1/1
  Integrator1/1 -> Sum2/1
  Sum2/1 -> f cos (rad)/1
  w/1 -> Sum1/1, Integrator1/1
  Kp1/1 -> Sum1/2
  Sum1/1 -> Integrator/1
  Trigonometric Function/1 -> Gain/1
  Gain/1 -> Poduct/2
  señal/1 -> Sum/1

== system Model_14Bus_Microgrid_R2018/Bus_14 /PLL/Pll3 ==
  note: error
  note: d'
  note: Fundamental
  note: fase
      | total
  note: fase de la señal
  note: adelanta 90
  note: Este PLL calcula la fase respecto a una onda coseno
  señal : Inport
  w : Inport  Port=2
  Gain : Gain  Gain=-1  SaturateOnIntegerOverflow=on  OutDataTypeStr=Inherit: Same as input  ParamDataTypeStr=Inherit: Same as input
  Integrator : Integrator  InitialCondition=2*pi*60
  Integrator1 : Integrator  InitialCondition=2*pi*60
  Integrator2 : Integrator
  K : Gain  Gain=100  SaturateOnIntegerOverflow=on  OutDataTypeStr=Inherit: Same as input  ParamDataTypeStr=Inherit: Same as input
  Kp : Gain  Gain=10  SaturateOnIntegerOverflow=on  OutDataTypeStr=Inherit: Same as input  ParamDataTypeStr=Inherit: Same as input
  Kp1 : Gain  Gain=10  SaturateOnIntegerOverflow=on  OutDataTypeStr=Inherit: Same as input  ParamDataTypeStr=Inherit: Same as input
  Poduct : Product  SaturateOnIntegerOverflow=on  OutDataTypeStr=Inherit: Same as first input
  Poduct1 : Product  SaturateOnIntegerOverflow=on  OutDataTypeStr=Inherit: Same as first input
  Poduct2 : Product  SaturateOnIntegerOverflow=on  OutDataTypeStr=Inherit: Same as first input
  Sum : Sum  Inputs=|+-  SaturateOnIntegerOverflow=on
  Sum1 : Sum  SaturateOnIntegerOverflow=on
  Sum2 : Sum  Inputs=|-+  SaturateOnIntegerOverflow=on
  Trigonometric Function : Trigonometry
  Trigonometric Function1 : Trigonometry  Operator=cos
  f cos (rad) : Outport
  wires:
  Sum/1 -> Poduct/1, Poduct1/1
  Poduct/1 -> Kp/1
  Kp/1 -> Kp1/1
  Poduct2/1 -> Sum/2
  Trigonometric Function1/1 -> Poduct1/2, Poduct2/1
  Poduct1/1 -> K/1
  K/1 -> Integrator2/1
  Integrator2/1 -> Poduct2/2
  Integrator/1 -> Trigonometric Function/1, Sum2/2, Trigonometric Function1/1
  Integrator1/1 -> Sum2/1
  Sum2/1 -> f cos (rad)/1
  w/1 -> Sum1/1, Integrator1/1
  Kp1/1 -> Sum1/2
  Sum1/1 -> Integrator/1
  Trigonometric Function/1 -> Gain/1
  Gain/1 -> Poduct/2
  señal/1 -> Sum/1

== system Model_14Bus_Microgrid_R2018/Bus_2/PLL/Pll1 ==
  note: error
  note: d'
  note: Fundamental
  note: fase
      | total
  note: fase de la señal
  note: adelanta 90
  note: Este PLL calcula la fase respecto a una onda coseno
  señal : Inport
  w : Inport  Port=2
  Gain : Gain  Gain=-1  SaturateOnIntegerOverflow=on  OutDataTypeStr=Inherit: Same as input  ParamDataTypeStr=Inherit: Same as input
  Integrator : Integrator  InitialCondition=2*pi*60
  Integrator1 : Integrator  InitialCondition=2*pi*60
  Integrator2 : Integrator
  K : Gain  Gain=100  SaturateOnIntegerOverflow=on  OutDataTypeStr=Inherit: Same as input  ParamDataTypeStr=Inherit: Same as input
  Kp : Gain  Gain=10  SaturateOnIntegerOverflow=on  OutDataTypeStr=Inherit: Same as input  ParamDataTypeStr=Inherit: Same as input
  Kp1 : Gain  Gain=10  SaturateOnIntegerOverflow=on  OutDataTypeStr=Inherit: Same as input  ParamDataTypeStr=Inherit: Same as input
  Poduct : Product  SaturateOnIntegerOverflow=on  OutDataTypeStr=Inherit: Same as first input
  Poduct1 : Product  SaturateOnIntegerOverflow=on  OutDataTypeStr=Inherit: Same as first input
  Poduct2 : Product  SaturateOnIntegerOverflow=on  OutDataTypeStr=Inherit: Same as first input
  Sum : Sum  Inputs=|+-  SaturateOnIntegerOverflow=on
  Sum1 : Sum  SaturateOnIntegerOverflow=on
  Sum2 : Sum  Inputs=|-+  SaturateOnIntegerOverflow=on
  Trigonometric Function : Trigonometry
  Trigonometric Function1 : Trigonometry  Operator=cos
  f cos (rad) : Outport
  wires:
  Sum/1 -> Poduct/1, Poduct1/1
  Poduct/1 -> Kp/1
  Kp/1 -> Kp1/1
  Poduct2/1 -> Sum/2
  Trigonometric Function1/1 -> Poduct1/2, Poduct2/1
  Poduct1/1 -> K/1
  K/1 -> Integrator2/1
  Integrator2/1 -> Poduct2/2
  Integrator/1 -> Trigonometric Function/1, Sum2/2, Trigonometric Function1/1
  Integrator1/1 -> Sum2/1
  Sum2/1 -> f cos (rad)/1
  w/1 -> Sum1/1, Integrator1/1
  Kp1/1 -> Sum1/2
  Sum1/1 -> Integrator/1
  Trigonometric Function/1 -> Gain/1
  Gain/1 -> Poduct/2
  señal/1 -> Sum/1

== system Model_14Bus_Microgrid_R2018/Bus_2/PLL/Pll2 ==
  note: error
  note: d'
  note: Fundamental
  note: fase
      | total
  note: fase de la señal
  note: adelanta 90
  note: Este PLL calcula la fase respecto a una onda coseno
  señal : Inport
  w : Inport  Port=2
  Gain : Gain  Gain=-1  SaturateOnIntegerOverflow=on  OutDataTypeStr=Inherit: Same as input  ParamDataTypeStr=Inherit: Same as input
  Integrator : Integrator  InitialCondition=2*pi*60
  Integrator1 : Integrator  InitialCondition=2*pi*60
  Integrator2 : Integrator
  K : Gain  Gain=100  SaturateOnIntegerOverflow=on  OutDataTypeStr=Inherit: Same as input  ParamDataTypeStr=Inherit: Same as input
  Kp : Gain  Gain=10  SaturateOnIntegerOverflow=on  OutDataTypeStr=Inherit: Same as input  ParamDataTypeStr=Inherit: Same as input
  Kp1 : Gain  Gain=10  SaturateOnIntegerOverflow=on  OutDataTypeStr=Inherit: Same as input  ParamDataTypeStr=Inherit: Same as input
  Poduct : Product  SaturateOnIntegerOverflow=on  OutDataTypeStr=Inherit: Same as first input
  Poduct1 : Product  SaturateOnIntegerOverflow=on  OutDataTypeStr=Inherit: Same as first input
  Poduct2 : Product  SaturateOnIntegerOverflow=on  OutDataTypeStr=Inherit: Same as first input
  Sum : Sum  Inputs=|+-  SaturateOnIntegerOverflow=on
  Sum1 : Sum  SaturateOnIntegerOverflow=on
  Sum2 : Sum  Inputs=|-+  SaturateOnIntegerOverflow=on
  Trigonometric Function : Trigonometry
  Trigonometric Function1 : Trigonometry  Operator=cos
  f cos (rad) : Outport
  wires:
  Sum/1 -> Poduct/1, Poduct1/1
  Poduct/1 -> Kp/1
  Kp/1 -> Kp1/1
  Poduct2/1 -> Sum/2
  Trigonometric Function1/1 -> Poduct1/2, Poduct2/1
  Poduct1/1 -> K/1
  K/1 -> Integrator2/1
  Integrator2/1 -> Poduct2/2
  Integrator/1 -> Trigonometric Function/1, Sum2/2, Trigonometric Function1/1
  Integrator1/1 -> Sum2/1
  Sum2/1 -> f cos (rad)/1
  w/1 -> Sum1/1, Integrator1/1
  Kp1/1 -> Sum1/2
  Sum1/1 -> Integrator/1
  Trigonometric Function/1 -> Gain/1
  Gain/1 -> Poduct/2
  señal/1 -> Sum/1

== system Model_14Bus_Microgrid_R2018/Bus_2/PLL/Pll3 ==
  note: error
  note: d'
  note: Fundamental
  note: fase
      | total
  note: fase de la señal
  note: adelanta 90
  note: Este PLL calcula la fase respecto a una onda coseno
  señal : Inport
  w : Inport  Port=2
  Gain : Gain  Gain=-1  SaturateOnIntegerOverflow=on  OutDataTypeStr=Inherit: Same as input  ParamDataTypeStr=Inherit: Same as input
  Integrator : Integrator  InitialCondition=2*pi*60
  Integrator1 : Integrator  InitialCondition=2*pi*60
  Integrator2 : Integrator
  K : Gain  Gain=100  SaturateOnIntegerOverflow=on  OutDataTypeStr=Inherit: Same as input  ParamDataTypeStr=Inherit: Same as input
  Kp : Gain  Gain=10  SaturateOnIntegerOverflow=on  OutDataTypeStr=Inherit: Same as input  ParamDataTypeStr=Inherit: Same as input
  Kp1 : Gain  Gain=10  SaturateOnIntegerOverflow=on  OutDataTypeStr=Inherit: Same as input  ParamDataTypeStr=Inherit: Same as input
  Poduct : Product  SaturateOnIntegerOverflow=on  OutDataTypeStr=Inherit: Same as first input
  Poduct1 : Product  SaturateOnIntegerOverflow=on  OutDataTypeStr=Inherit: Same as first input
  Poduct2 : Product  SaturateOnIntegerOverflow=on  OutDataTypeStr=Inherit: Same as first input
  Sum : Sum  Inputs=|+-  SaturateOnIntegerOverflow=on
  Sum1 : Sum  SaturateOnIntegerOverflow=on
  Sum2 : Sum  Inputs=|-+  SaturateOnIntegerOverflow=on
  Trigonometric Function : Trigonometry
  Trigonometric Function1 : Trigonometry  Operator=cos
  f cos (rad) : Outport
  wires:
  Sum/1 -> Poduct/1, Poduct1/1
  Poduct/1 -> Kp/1
  Kp/1 -> Kp1/1
  Poduct2/1 -> Sum/2
  Trigonometric Function1/1 -> Poduct1/2, Poduct2/1
  Poduct1/1 -> K/1
  K/1 -> Integrator2/1
  Integrator2/1 -> Poduct2/2
  Integrator/1 -> Trigonometric Function/1, Sum2/2, Trigonometric Function1/1
  Integrator1/1 -> Sum2/1
  Sum2/1 -> f cos (rad)/1
  w/1 -> Sum1/1, Integrator1/1
  Kp1/1 -> Sum1/2
  Sum1/1 -> Integrator/1
  Trigonometric Function/1 -> Gain/1
  Gain/1 -> Poduct/2
  señal/1 -> Sum/1

== system Model_14Bus_Microgrid_R2018/Bus_3/PLL/Pll1 ==
  note: error
  note: d'
  note: Fundamental
  note: fase
      | total
  note: fase de la señal
  note: adelanta 90
  note: Este PLL calcula la fase respecto a una onda coseno
  señal : Inport
  w : Inport  Port=2
  Gain : Gain  Gain=-1  SaturateOnIntegerOverflow=on  OutDataTypeStr=Inherit: Same as input  ParamDataTypeStr=Inherit: Same as input
  Integrator : Integrator  InitialCondition=2*pi*60
  Integrator1 : Integrator  InitialCondition=2*pi*60
  Integrator2 : Integrator
  K : Gain  Gain=100  SaturateOnIntegerOverflow=on  OutDataTypeStr=Inherit: Same as input  ParamDataTypeStr=Inherit: Same as input
  Kp : Gain  Gain=10  SaturateOnIntegerOverflow=on  OutDataTypeStr=Inherit: Same as input  ParamDataTypeStr=Inherit: Same as input
  Kp1 : Gain  Gain=10  SaturateOnIntegerOverflow=on  OutDataTypeStr=Inherit: Same as input  ParamDataTypeStr=Inherit: Same as input
  Poduct : Product  SaturateOnIntegerOverflow=on  OutDataTypeStr=Inherit: Same as first input
  Poduct1 : Product  SaturateOnIntegerOverflow=on  OutDataTypeStr=Inherit: Same as first input
  Poduct2 : Product  SaturateOnIntegerOverflow=on  OutDataTypeStr=Inherit: Same as first input
  Sum : Sum  Inputs=|+-  SaturateOnIntegerOverflow=on
  Sum1 : Sum  SaturateOnIntegerOverflow=on
  Sum2 : Sum  Inputs=|-+  SaturateOnIntegerOverflow=on
  Trigonometric Function : Trigonometry
  Trigonometric Function1 : Trigonometry  Operator=cos
  f cos (rad) : Outport
  wires:
  Sum/1 -> Poduct/1, Poduct1/1
  Poduct/1 -> Kp/1
  Kp/1 -> Kp1/1
  Poduct2/1 -> Sum/2
  Trigonometric Function1/1 -> Poduct1/2, Poduct2/1
  Poduct1/1 -> K/1
  K/1 -> Integrator2/1
  Integrator2/1 -> Poduct2/2
  Integrator/1 -> Trigonometric Function/1, Sum2/2, Trigonometric Function1/1
  Integrator1/1 -> Sum2/1
  Sum2/1 -> f cos (rad)/1
  w/1 -> Sum1/1, Integrator1/1
  Kp1/1 -> Sum1/2
  Sum1/1 -> Integrator/1
  Trigonometric Function/1 -> Gain/1
  Gain/1 -> Poduct/2
  señal/1 -> Sum/1
